simulink model "vtol_att_control"  (R2021a)
settings: Solver=FixedStepAuto  StartTime=0.0  StopTime=10.0  RelTol=1e-3
undefined symbols (not defined in the file): FW_PSP_OFF, MPC_XY_CRUISE, VT_ARSP_BLEND, VT_ARSP_TRANS, VT_B_DEC_FF, VT_B_DEC_I, VT_B_DEC_MSS, VT_B_REV_DEL, VT_B_REV_OUT, VT_B_TRANS_DUR, VT_B_TRANS_RAMP, VT_ELEV_MC_LOCK, VT_F_TRANS_THR, VT_FW_ALT_ERR, VT_FW_MIN_ALT, VT_FW_QC_P, VT_FW_QC_R, VT_PSHER_RMP_DT, VT_TRANS_MIN_TM, VT_TRANS_TIMEOUT
settings Model: DataDictionary=px4_dict.sldd  Creator=DELL  LastModifiedBy=DELL
settings OptimizationCC: GainParamInheritBuiltInType=on  UseFloatMulNetSlope=on  DefaultUnderspecifiedDataType=single  OptimizeBlockIOStorage=off  EnhancedBackFolding=on  PassReuseOutputArgsAs=Individual arguments  NoFixptDivByZeroProtection=on  EfficientFloat2IntCast=on  LifeSpan=1  OptimizeBlockOrder=speed  DifferentSizesBufferReuse=on  EfficientTunableParamExpr=on
settings DebuggingCC: ParameterTunabilityLossMsg=error
settings HardwareCC: ProdBitPerPointer=32  ProdBitPerSizeT=32  ProdBitPerPtrDiffT=32  ProdLargestAtomicInteger=Long  ProdLargestAtomicFloat=Double  ProdWordSize=32  ProdLongLongMode=on  ProdHWDeviceType=ARM Compatible->ARM Cortex-M
settings SFSimCC: MATLABDynamicMemAlloc=off
settings RTWCC: SystemTargetFile=ert.tlc  TemplateMakefile=ert_default_tmf  GenerateReport=on  LaunchReport=on  GenerateWebview=on  GenerateCodeMetricsReport=on
settings CodeAppCC: ForceParamTrailComments=on  IgnoreCustomStorageClasses=off  MaxIdLength=64  OperatorAnnotations=on  SimulinkDataObjDesc=on  SFDataObjDesc=on  MATLABFcnDesc=on  CustomSymbolStrGlobalVar=rt$N$M  CustomSymbolStrType=$N$M  CustomSymbolStrFcn=$N$M$F  CustomSymbolStrMacro=$N$M  InsertBlockDesc=on  SimulinkBlockComments=off  StateflowObjectComments=on
settings ERTTargetCC: TargetLangStandard=C99 (ISO)  GenerateSampleERTMain=on  CombineSignalStateStructs=on  SupportComplex=off  SupportNonInlinedSFcns=on  SupportVariableSizeSignals=on  RTWCAPISignals=on  RTWCAPIParams=on  RTWCAPIStates=on  ERTCustomFileTemplate=example_file_process.tlc  ERTFilePackagingFormat=CompactWithDataFile  IndentSize=4  MaxLineWidth=256

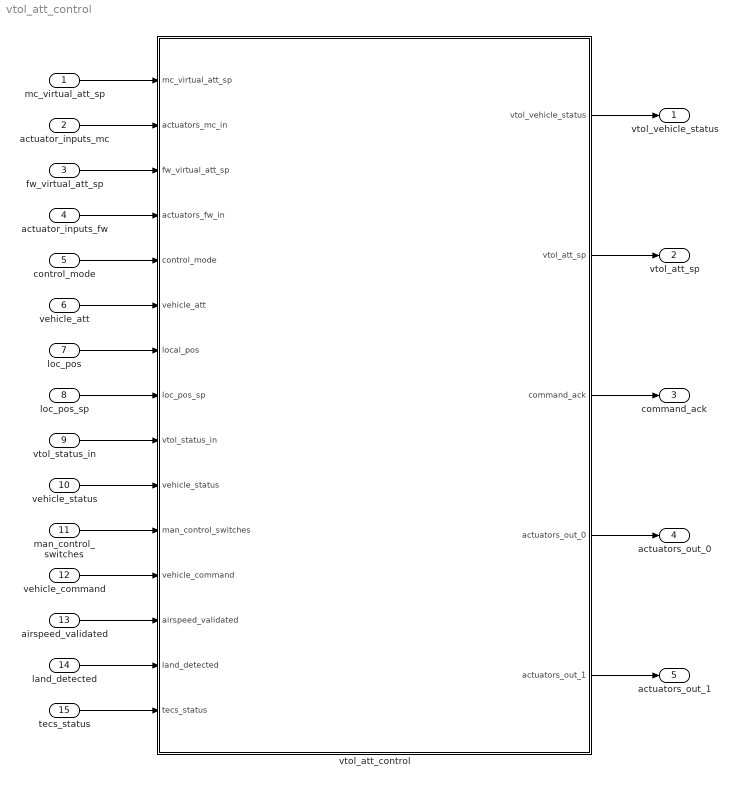
== system vtol_att_control ==
  mc_virtual_att_sp : Inport  OutDataTypeStr=Bus: px4_vehicle_attitude_setpoint  BusOutputAsStruct=on
  actuator_inputs_mc : Inport  Port=2  OutDataTypeStr=Bus: px4_actuator_controls_0  BusOutputAsStruct=on
  fw_virtual_att_sp : Inport  Port=3  OutDataTypeStr=Bus: px4_vehicle_attitude_setpoint  BusOutputAsStruct=on
  actuator_inputs_fw : Inport  Port=4  OutDataTypeStr=Bus: px4_actuator_controls_0  BusOutputAsStruct=on
  control_mode : Inport  Port=5  OutDataTypeStr=Bus: px4_vehicle_control_mode  BusOutputAsStruct=on
  vehicle_att : Inport  Port=6  OutDataTypeStr=Bus: px4_vehicle_attitude  BusOutputAsStruct=on
  loc_pos : Inport  Port=7  OutDataTypeStr=Bus: px4_vehicle_local_position  BusOutputAsStruct=on
  loc_pos_sp : Inport  Port=8  OutDataTypeStr=Bus: px4_vehicle_local_position_setpoint  BusOutputAsStruct=on
  vtol_status_in : Inport  Port=9  OutDataTypeStr=Bus: px4_vtol_vehicle_status  BusOutputAsStruct=on
  vehicle_status : Inport  Port=10  OutDataTypeStr=Bus: px4_vehicle_status  BusOutputAsStruct=on
  man_control_switches : Inport  Port=11  OutDataTypeStr=Bus: px4_manual_control_switches  BusOutputAsStruct=on
  vehicle_command : Inport  Port=12  OutDataTypeStr=Bus: px4_vehicle_command  BusOutputAsStruct=on
  airspeed_validated : Inport  Port=13  OutDataTypeStr=Bus: px4_airspeed_validated  BusOutputAsStruct=on
  land_detected : Inport  Port=14  OutDataTypeStr=Bus: px4_vehicle_land_detected  BusOutputAsStruct=on
  tecs_status : Inport  Port=15  OutDataTypeStr=Bus: px4_tecs_status  BusOutputAsStruct=on
  vtol_att_control : Stateflow chart  TreatAsAtomicUnit=on
  vtol_vehicle_status : Outport  OutDataTypeStr=Bus: px4_vtol_vehicle_status
  vtol_att_sp : Outport  Port=2  OutDataTypeStr=Bus: px4_vehicle_attitude_setpoint
  command_ack : Outport  Port=3  OutDataTypeStr=Bus: px4_vehicle_command_ack
  actuators_out_0 : Outport  Port=4  OutDataTypeStr=Bus: px4_actuator_controls_0
  actuators_out_1 : Outport  Port=5  OutDataTypeStr=Bus: px4_actuator_controls
  wires:
  fw_virtual_att_sp/1 -> vtol_att_control/3(fw_virtual_att_sp)
  actuator_inputs_mc/1 -> vtol_att_control/2(actuators_mc_in)
  vehicle_att/1 -> vtol_att_control/6(vehicle_att)
  loc_pos/1 -> vtol_att_control/7(local_pos)
  vehicle_command/1 -> vtol_att_control/12(vehicle_command)
  airspeed_validated/1 -> vtol_att_control/13(airspeed_validated)
  control_mode/1 -> vtol_att_control/5(control_mode)
  mc_virtual_att_sp/1 -> vtol_att_control/1(mc_virtual_att_sp)
  vtol_att_control/4(actuators_out_0) -> actuators_out_0/1
  loc_pos_sp/1 -> vtol_att_control/8(loc_pos_sp)
  land_detected/1 -> vtol_att_control/14(land_detected)
  actuator_inputs_fw/1 -> vtol_att_control/4(actuators_fw_in)
  tecs_status/1 -> vtol_att_control/15(tecs_status)
  vtol_att_control/2(vtol_att_sp) -> vtol_att_sp/1
  vtol_att_control/3(command_ack) -> command_ack/1
  vtol_att_control/1(vtol_vehicle_status) -> vtol_vehicle_status/1
  vtol_status_in/1 -> vtol_att_control/9(vtol_status_in)
  vehicle_status/1 -> vtol_att_control/10(vehicle_status)
  vtol_att_control/5(actuators_out_1) -> actuators_out_1/1
  man_control_switches/1 -> vtol_att_control/11(man_control_switches)

== stateflow chart vtol_att_control/vtol_att_control ==
  state vehicle_cmd_poll [parallel]
    settings: executionOrder=1
    state DO_VTOL_TRANSITION
      en:
      result = PX4_VEHICLE_COMMAND_ACK.VEHICLE_RESULT_ACCEPTED;
      % 在自动起飞阶段、或者在land或者RTL模式下拒绝从RW转换到FW
      if (vehicle_command.command == PX4_VEHICLE_COMMAND.VEHICLE_CMD_DO_VTOL_TRANSITION)
      if (vehicle_status.nav_state == PX4_VEHICLE_STATUS.NAVIGATION_STATE_AUTO_TAKEOFF || ...
      (vehicle_status.vehicle_type == PX4_VEHICLE_STATUS.VEHICLE_TYPE_ROTARY_WING && ...
      vehicle_status.nav_state == PX4_VEHICLE_STATUS.NAVIGATION_STATE_AUTO_LAND || ...
      vehicle_status.nav_state == PX4_VEHICLE_STATUS.NAVIGATION_STATE_AUTO_RTL))
      result = PX4_VEHICLE_COMMAND_ACK.VEHICLE_RESULT_TEMPORARILY_REJECTED;
      else
      transition_command_ = int8(vehicle_command.param1 + 0.5);
      if (isfinite(vehicle_command.param2))
      immediate_transition_ = int8(vehicle_command.param2 + 0.5)
      else
      immediate_transition_ = int8(false);
      end
      end
      end
      % 如果command是来自外部的，不是飞机自己发布的
      if (vehicle_command.from_external)
      command_ack.timestamp = uint64(getSimulationTime * 1e+6); % 单位：us
      command_ack.command = vehicle_command.command;
      command_ack.result = uint8(result);
      command_ack.target_system = vehicle_command.source_system;
      command_ack.target_component = vehicle_command.source_component;
      end
    state NONE
    state KEEP_IN_MC
      en:
      transition_command_ = int8(PX4_VTOL_VEHICLE_STATUS.VEHICLE_VTOL_STATE_MC);
    state KEEP_IN_FW
      en:
      transition_command_ = int8(PX4_VTOL_VEHICLE_STATUS.VEHICLE_VTOL_STATE_FW);
    state TRANSITION_TO_MC
      en:
      % We want to make sure that a mode change (manual>auto) during the back transition
      % doesn't result in an unsafe state. This prevents the instant fall back to
      % fixed-wing on the switch from manual to auto.
      % 飞机本来是在从固定翼过渡到旋翼模式的时候，如果接管，那么直接变成旋翼模式
      transition_command_ = int8(PX4_VTOL_VEHICLE_STATUS.VEHICLE_VTOL_STATE_MC);
    state NONE1
    (default) -> (junction 580)
    vehicle_cmd_poll -> (junction 580) [order 1] : % 轮询是否有开启转换的指令
        | [hasChanged(vehicle_command.timestamp)]
    (junction 580) -> DO_VTOL_TRANSITION [order 1] : [vehicle_command.command == PX4_VEHICLE_COMMAND.VEHICLE_CMD_DO_VTOL_TRANSITION]
    (junction 580) -> (junction 581) [order 2]
    (junction 581) -> NONE
    vehicle_cmd_poll -> (junction 582) [order 2] : % reset transition command if not auto control
        | [control_mode.flag_control_manual_enabled == true]
    (junction 582) -> KEEP_IN_MC [order 1] : % vtol_mode_ == mode::ROTARY_WING
        | [vtol_mode_ == uint8(3)]
    (junction 582) -> (junction 583) [order 2]
    (junction 583) -> KEEP_IN_FW [order 1] : % vtol_mode_ == mode::FIXED_WING
        | [vtol_mode_ == uint8(4)]
    (junction 583) -> (junction 584) [order 2]
    (junction 584) -> TRANSITION_TO_MC [order 1] : % mode::TRANSITION_TO_MC
        | [vtol_mode_ == uint8(2)]
    (junction 584) -> (junction 585) [order 2]
    (junction 585) -> NONE1
  state vtol_state_flow [parallel]
    settings: executionOrder=2
    state MC_MODE_
      en:
      vtol_schedule_.flight_mode = uint8(PX4_VTOL_MODE.MC_MODE);
      vtol_mode_ = uint8(PX4_VTOL_MODETYPE.ROTARY_WING);
      % 转换失败保护或者没有开启过渡到固定翼的开关，那么启用旋翼模式
      if (vtol_status_in.vtol_transition_failsafe || ~vtol_state_flow.is_fixed_wing_requested)
      pusher_throttle_ = single(0.0);
      reverse_output_ = single(0.0);
      % reset failsafe when FW is no longer requested
      % 转换失败后，如果转换通道还在保持请求转换到固定翼，那么vtol_transition_failsafe标志位保持置位为true
      % 转换失败后，用户不再请求转换到固定翼，vtol_transition_failsafe标志位重置为false
      if (vtol_status_in.vtol_transition_failsafe && ~vtol_state_flow.is_fixed_wing_requested)
      vtol_vehicle_status.vtol_transition_failsafe = false;
      end
      end
      % 正常进入，关闭固定翼转换
      en,du:
      mc_weight_ = single(1.0);
      pusher_throttle_ = single(0.0);
      reverse_output_ = single(0.0);
      %
      % update mc mode
      vtol_vehicle_status.vtol_in_rw_mode = true;
      vtol_vehicle_status.vtol_in_trans_mode = false;
      vtol_vehicle_status.in_transition_to_fw = false;
      if (~flag_idle_mc_)
      % flag_idle_mc_ = set_idle_mc();
      end
      % resetAccelToPitchPitchIntegrator
      accel_to_pitch_integ_ = single(0.0);
      % mode_action.set_all_motor_state(PX4_MOTOR_STATE.ENABLED, 0);
      mc_roll_weight_ = 1.0;
      mc_pitch_weight_ = 1.0;
      mc_yaw_weight_ = 1.0;
      mc_throttle_weight_ = 1.0;
      % pusher_assist()没看懂这个函数
      % publish actuators_out_0
      vtol_att_sp = mc_virtual_att_sp;
      elevon_lock = (VT_ELEV_MC_LOCK == 1);
      now_us = uint64(getSimulationTime * 1e+6);
      actuators_out_0.timestamp = now_us;
      actuators_out_0.timestamp_sample = actuators_mc_in.timestamp_sample;
      actuators_out_0.control(PX4_ACTUATOR_CONTROLS.INDEX_ROLL) = actuators_mc_in.control(PX4_ACTUATOR_CONTROLS.INDEX_ROLL);
      actuators_out_0.control(PX4_ACTUATOR_CONTROLS.INDEX_PITCH) = actuators_mc_in.control(PX4_ACTUATOR_CONTROLS.INDEX_PITCH);
      actuators_out_0.control(PX4_ACTUATOR_CONTROLS.INDEX_YAW) = actuators_mc_in.control(PX4_ACTUATOR_CONTROLS.INDEX_YAW);
      actuators_out_0.control(PX4_ACTUATOR_CONTROLS.INDEX_THROTTLE) = actuators_mc_in.control(PX4_ACTUATOR_CONTROLS.INDEX_THROTTLE);
      actuators_out_0.control(PX4_ACTUATOR_CONTROLS.INDEX_LANDING_GEAR) = actuators_mc_in.control(PX4_ACTUATOR_CONTROLS.INDEX_LANDING_GEAR);
      % publish actuators_out_1
      actuators_out_1.timestamp = now_us;
      actuators_out_1.timestamp_sample = actuators_mc_in.timestamp_sample;
      actuators_out_1.control(PX4_ACTUATOR_CONTROLS.INDEX_ROLL) = single(~elevon_lock) * actuators_fw_in.control(PX4_ACTUATOR_CONTROLS.INDEX_ROLL);
      actuators_out_1.control(PX4_ACTUATOR_CONTROLS.INDEX_PITCH) = single(~elevon_lock) * actuators_fw_in.control(PX4_ACTUATOR_CONTROLS.INDEX_PITCH);
      actuators_out_1.control(PX4_ACTUATOR_CONTROLS.INDEX_YAW) = single(0.0);
      actuators_out_1.control(PX4_ACTUATOR_CONTROLS.INDEX_THROTTLE) = pusher_throttle_;
      actuators_out_1.control(PX4_ACTUATOR_CONTROLS.INDEX_FLAPS) = single(0.0);
      actuators_out_1.control(PX4_ACTUATOR_CONTROLS.INDEX_AIRBRAKES) = single(0.0);
    state TRANSITION_TO_FW_
      en:
      vtol_schedule_.transition_start = uint64(getSimulationTime) * 1e+6; % 单位：us
      vtol_schedule_.flight_mode = uint8(PX4_VTOL_MODE.TRANSITION_TO_FW);
      vtol_mode_ = uint8(PX4_VTOL_MODETYPE.TRANSITION_TO_FW);
      % 飞机当前正处于过渡到固定翼的阶段
      en,du:
      % 计算转换条件（看是否能转换到固定翼阶段）
      time_since_trans_start_ = single(elapsed(sec));
      % update transition to fw
      vtol_vehicle_status.vtol_in_trans_mode = true;
      vtol_vehicle_status.vtol_in_rw_mode = true; % making mc attitude controller work during transition
      vtol_vehicle_status.in_transition_to_fw = (vtol_mode_ == PX4_VTOL_MODETYPE.TRANSITION_TO_FW);
      %
      if ((flag_was_in_trans_mode_ == false) || hasChanged(mc_virtual_att_sp.timestamp) || hasChanged(fw_virtual_att_sp.timestamp))
      vtol_state_flow.check_quadchute_condition;
      % copy virtual attitude setpoint to real attitude setpoint
      vtol_att_sp = mc_virtual_att_sp;
      transition_to_fw;
      % publish actuators_out_0
      now_us = uint64(getSimulationTime * 1e+6);
      actuators_out_0.timestamp = now_us;
      actuators_out_0.timestamp_sample = actuators_mc_in.timestamp_sample;
      actuators_out_0.control(PX4_ACTUATOR_CONTROLS.INDEX_ROLL) = actuators_mc_in.control(PX4_ACTUATOR_CONTROLS.INDEX_ROLL) * mc_roll_weight_;
      actuators_out_0.control(PX4_ACTUATOR_CONTROLS.INDEX_PITCH) = actuators_mc_in.control(PX4_ACTUATOR_CONTROLS.INDEX_PITCH) * mc_pitch_weight_;
      actuators_out_0.control(PX4_ACTUATOR_CONTROLS.INDEX_YAW) = actuators_mc_in.control(PX4_ACTUATOR_CONTROLS.INDEX_YAW) * mc_yaw_weight_;
      actuators_out_0.control(PX4_ACTUATOR_CONTROLS.INDEX_THROTTLE) = actuators_mc_in.control(PX4_ACTUATOR_CONTROLS.INDEX_THROTTLE) * mc_throttle_weight_;
      actuators_out_0.control(PX4_ACTUATOR_CONTROLS.INDEX_LANDING_GEAR) = single(0.0);
      % publish actuators_out_1
      actuators_out_1.timestamp = now_us;
      actuators_out_1.timestamp_sample = actuators_mc_in.timestamp_sample;
      actuators_out_1.control(PX4_ACTUATOR_CONTROLS.INDEX_ROLL) = actuators_fw_in.control(PX4_ACTUATOR_CONTROLS.INDEX_ROLL);
      actuators_out_1.control(PX4_ACTUATOR_CONTROLS.INDEX_PITCH) = actuators_fw_in.control(PX4_ACTUATOR_CONTROLS.INDEX_PITCH);
      actuators_out_1.control(PX4_ACTUATOR_CONTROLS.INDEX_YAW) = actuators_fw_in.control(PX4_ACTUATOR_CONTROLS.INDEX_YAW);
      actuators_out_1.control(PX4_ACTUATOR_CONTROLS.INDEX_THROTTLE) = pusher_throttle_;
      actuators_out_1.control(PX4_ACTUATOR_CONTROLS.INDEX_FLAPS) = actuators_fw_in.control(PX4_ACTUATOR_CONTROLS.INDEX_FLAPS);
      actuators_out_1.control(PX4_ACTUATOR_CONTROLS.INDEX_AIRBRAKES) = reverse_output_;
      end
    state FW_MODE_
      en:
      trans_finished_ts_ = uint64(getSimulationTime * 1e+6); % 单位：us
      vtol_schedule_.flight_mode = uint8(PX4_VTOL_MODE.FW_MODE);
      vtol_mode_ = uint8(PX4_VTOL_MODETYPE.FIXED_WING);
      % 正常情况下，进入固定翼模式后，保持该模式飞行
      en,du:
      mc_weight_ = single(0.0);
      vtol_vehicle_status.vtol_in_rw_mode = false;
      vtol_vehicle_status.vtol_in_trans_mode = false;
      vtol_vehicle_status.in_transition_to_fw = false;
      % 更新固定翼状态
      if (hasChanged(fw_virtual_att_sp.timestamp))
      if (flag_idle_mc_)
      % flag_idle_mc_ = ~set_idle_fw();
      end
      % resetAccelToPitchPitchIntegrator
      accel_to_pitch_integ_ = single(0.0);
      % set_alternate_motor_state(PX4_MOTOR_STATE.DISABLED, 0);
      mc_roll_weight_ = single(0.0);
      mc_pitch_weight_ = single(0.0);
      mc_yaw_weight_ = single(0.0);
      %
      % publish
      % copy virtual attitude setpoint to real attitude setpoint
      vtol_att_sp = fw_virtual_att_sp;
      % 在转换成固定翼完成后，tecs还未发布tecs_status的topic，暂时“认为”tecs没有running
      if (tecs_status.timestamp < trans_finished_ts_)
      tecs_running_ = false;
      elseif (~tecs_running_)
      tecs_running_ = true;
      tecs_running_ts = uint64(getSimulationTime) * 1e+6; % 单位：us
      end
      % 如果tecs没有运行，或在手动控制高度的情况下，tecs发布了但控制器还没运行完，保持pusher_throttle_不变
      if((~tecs_running_ || (tecs_running_ && fw_virtual_att_sp.timestamp <= tecs_running_ts)) && control_mode.flag_control_altitude_enabled)
      % keep thrust from transition
      vtol_att_sp.thrust_body(1) = pusher_throttle_;
      end
      vtol_state_flow.check_quadchute_condition;
      % publish actuators_out_0
      actuators_out_0.timestamp = now_us;
      actuators_out_0.timestamp_sample = actuators_mc_in.timestamp_sample;
      actuators_out_0.control(PX4_ACTUATOR_CONTROLS.INDEX_ROLL) = single(0.0);
      actuators_out_0.control(PX4_ACTUATOR_CONTROLS.INDEX_PITCH) = single(0.0);
      actuators_out_0.control(PX4_ACTUATOR_CONTROLS.INDEX_YAW) = single(0.0);
      actuators_out_0.control(PX4_ACTUATOR_CONTROLS.INDEX_THROTTLE) = single(0.0);
      actuators_out_0.control(PX4_ACTUATOR_CONTROLS.INDEX_LANDING_GEAR) = single(0.0);
      % publish actuators_out_1
      actuators_out_1.timestamp = now_us;
      actuators_out_1.timestamp_sample = actuators_mc_in.timestamp_sample;
      actuators_out_1.control(PX4_ACTUATOR_CONTROLS.INDEX_ROLL) = actuators_fw_in.control(PX4_ACTUATOR_CONTROLS.INDEX_ROLL);
      actuators_out_1.control(PX4_ACTUATOR_CONTROLS.INDEX_PITCH) = actuators_fw_in.control(PX4_ACTUATOR_CONTROLS.INDEX_PITCH);
      actuators_out_1.control(PX4_ACTUATOR_CONTROLS.INDEX_YAW) = actuators_fw_in.control(PX4_ACTUATOR_CONTROLS.INDEX_YAW);
      actuators_out_1.control(PX4_ACTUATOR_CONTROLS.INDEX_THROTTLE) = actuators_fw_in.control(PX4_ACTUATOR_CONTROLS.INDEX_THROTTLE);
      actuators_out_1.control(PX4_ACTUATOR_CONTROLS.INDEX_FLAPS) = actuators_fw_in.control(PX4_ACTUATOR_CONTROLS.INDEX_FLAPS);
      actuators_out_1.control(PX4_ACTUATOR_CONTROLS.INDEX_AIRBRAKES) = actuators_fw_in.control(PX4_ACTUATOR_CONTROLS.INDEX_LANDING_GEAR);
      end
    state TRANSITION_TO_MC_
      en:
      % 没有请求转换到固定翼模式，就会切回旋翼模式
      if (~vtol_state_flow.is_fixed_wing_requested)
      % 单位：us
      vtol_schedule_.transition_start = uint64(getSimulationTime * 1e+6);
      reverse_output_ = constrain(VT_B_REV_OUT, 0.0, 1.0);
      end
      % 固定翼转多旋翼
      en,du:
      % 计算转换成旋翼模式失败的条件
      time_since_trans_start_ = single(elapsed(sec));
      R_to_body = quat_to_dcm(vehicle_att.q);
      vel = R_to_body * [local_pos.vx; local_pos.vy; local_pos.vz];
      x_vel = vel(1);
      % 更新过渡转换，转换到多旋翼模式
      vtol_vehicle_status.vtol_in_trans_mode = true;
      vtol_vehicle_status.vtol_in_rw_mode = true;
      vtol_vehicle_status.in_transition_to_fw = (vtol_mode_ == PX4_VTOL_MODETYPE.TRANSITION_TO_FW);
      transition_to_mc();
      % publish actuators_out_0
      now_us = uint64(getSimulationTime * 1e+6);
      actuators_out_0.timestamp = now_us;
      actuators_out_0.timestamp_sample = actuators_mc_in.timestamp_sample;
      actuators_out_0.control(PX4_ACTUATOR_CONTROLS.INDEX_ROLL) = actuators_mc_in.control(PX4_ACTUATOR_CONTROLS.INDEX_ROLL) * mc_roll_weight_;
      actuators_out_0.control(PX4_ACTUATOR_CONTROLS.INDEX_PITCH) = actuators_mc_in.control(PX4_ACTUATOR_CONTROLS.INDEX_PITCH) * mc_pitch_weight_;
      actuators_out_0.control(PX4_ACTUATOR_CONTROLS.INDEX_YAW) = actuators_mc_in.control(PX4_ACTUATOR_CONTROLS.INDEX_YAW) * mc_yaw_weight_;
      actuators_out_0.control(PX4_ACTUATOR_CONTROLS.INDEX_THROTTLE) = actuators_mc_in.control(PX4_ACTUATOR_CONTROLS.INDEX_THROTTLE) * mc_throttle_weight_;
      actuators_out_0.control(PX4_ACTUATOR_CONTROLS.INDEX_LANDING_GEAR) = single(0.0);
      % publish actuators_out_1
      actuators_out_1.timestamp = now_us;
      actuators_out_1.timestamp_sample = actuators_mc_in.timestamp_sample;
      actuators_out_1.control(PX4_ACTUATOR_CONTROLS.INDEX_ROLL) = actuators_fw_in.control(PX4_ACTUATOR_CONTROLS.INDEX_ROLL);
      actuators_out_1.control(PX4_ACTUATOR_CONTROLS.INDEX_PITCH) = actuators_fw_in.control(PX4_ACTUATOR_CONTROLS.INDEX_PITCH);
      actuators_out_1.control(PX4_ACTUATOR_CONTROLS.INDEX_YAW) = actuators_fw_in.control(PX4_ACTUATOR_CONTROLS.INDEX_YAW);
      actuators_out_1.control(PX4_ACTUATOR_CONTROLS.INDEX_THROTTLE) = pusher_throttle_;
      actuators_out_1.control(PX4_ACTUATOR_CONTROLS.INDEX_FLAPS) = actuators_fw_in.control(PX4_ACTUATOR_CONTROLS.INDEX_FLAPS);
      actuators_out_1.control(PX4_ACTUATOR_CONTROLS.INDEX_AIRBRAKES) = reverse_output_;
    (default) -> MC_MODE_
    MC_MODE_ -> TRANSITION_TO_FW_ : % 请求转换到固定翼模式
        | [is_fixed_wing_requested()]
    TRANSITION_TO_FW_ -> FW_MODE_ [order 1] : % 满足转换时间且空速大于转换的阈值
        | % 或未解锁或飞机在地面
        | [((time_since_trans_start_ > VT_TRANS_MIN_TM) && ...
        | isfinite(airspeed_validated.calibrated_airspeed_m_s) && ...
        | (airspeed_validated.calibrated_airspeed_m_s >= VT_TRANS_MIN_TM)) || ...
        | (~control_mode.flag_armed || land_detected.landed)]
    TRANSITION_TO_FW_ -> MC_MODE_ [order 2] : % 没有请求转换到固定翼模式
        | % 或者转换失败
        | [~is_fixed_wing_requested() || ...
        | vtol_status_in.vtol_transition_failsafe]
    (junction 533) -> MC_MODE_
    TRANSITION_TO_MC_ -> TRANSITION_TO_FW_ [order 1] : % 请求转换到固定翼模式
        | [is_fixed_wing_requested()]
    FW_MODE_ -> (junction 537)
    TRANSITION_TO_MC_ -> (junction 533) [order 2] : % 转换超时，或者前向速度低于旋翼的巡航速
        | % 或未解锁或飞机在地面
        | [(time_since_trans_start_ > VT_B_TRANS_DUR) || ...
        |  (local_pos.v_xy_valid && x_vel <= MPC_XY_CRUISE) || ...
        |  (~control_mode.flag_armed || land_detected.landed)]
    (junction 537) -> TRANSITION_TO_MC_ : % 没有请求转换到固定翼模式
        | [~is_fixed_wing_requested() || ...
        | (vtol_schedule_.flight_mode == uint8(PX4_VTOL_MODE.TRANSITION_TO_MC))]
  data: result local Enum: PX4_VEHICLE_COMMAND_ACK size=1; to_fw function_output; elevon_lock local boolean size=1 =false; tecs_running_ts local uint64 size=1 =uint64(0); R_to_body local single size=[3 3]; vel local single size=[3 1]; x_vel local single size=1 =single(0.0); quadchute_command_treated_ local boolean size=1 =false; tecs_running_ local boolean size=1 =false; ra_hrate_ local single size=1 =single(0.0); ra_hrate_sp_ local single size=1 =single(0.0); now_us local uint64 size=1 =uint64(0); mc_virtual_att_sp input Bus: px4_vehicle_attitude_setpoint size=1; actuators_mc_in input Bus: px4_actuator_controls_0 size=1; fw_virtual_att_sp input Bus: px4_vehicle_attitude_setpoint size=1; actuators_fw_in input Bus: px4_actuator_controls_0 size=1; control_mode input Bus: px4_vehicle_control_mode size=1; vehicle_att input Bus: px4_vehicle_attitude size=1; local_pos input Bus: px4_vehicle_local_position size=1; loc_pos_sp input Bus: px4_vehicle_local_position_setpoint size=1; vtol_status_in input Bus: px4_vtol_vehicle_status size=1; vehicle_status input Bus: px4_vehicle_status size=1; man_control_switches input Bus: px4_manual_control_switches size=1; vehicle_command input Bus: px4_vehicle_command size=1; pusher_throttle_ local single size=1 =single(0.0); reverse_output_ local single size=1 =single(0.0); vtol_vehicle_status output Bus: px4_vtol_vehicle_status size=1; vtol_schedule_ local Bus: px4_vtol_schedule size=1; mc_weight_ local single size=1 =single(1.0); VT_B_REV_OUT parameter size=1; airspeed_validated input Bus: px4_airspeed_validated size=1; VT_TRANS_MIN_TM parameter size=1; VT_ARSP_TRANS parameter size=1; trans_finished_ts_ local uint64 size=1 =uint64(0); vtol_mode_ local uint8 size=1 =uint8(3); transition_command_ local int8 size=1 =int8(3); VT_PSHER_RMP_DT parameter size=1; VT_F_TRANS_THR parameter size=1; VT_ARSP_BLEND parameter size=1; vtol_att_sp output Bus: px4_vehicle_attitude_setpoint size=1; command_ack output Bus: px4_vehicle_command_ack size=1; FW_PSP_OFF parameter size=1; VT_TRANS_TIMEOUT parameter size=1; VT_B_REV_DEL parameter size=1; VT_B_TRANS_RAMP parameter size=1; flag_idle_mc_ local boolean size=1 =false; mc_roll_weight_ local single size=1 =single(0.0); mc_pitch_weight_ local single size=1 =single(0.0); mc_yaw_weight_ local single size=1 =single(0.0); mc_throttle_weight_ local single size=1 =single(0.0); VT_B_DEC_MSS parameter size=1; VT_B_DEC_FF parameter size=1; accel_to_pitch_integ_ local single size=1 =single(0.0); VT_B_DEC_I parameter size=1; actuators_out_0 output Bus: px4_actuator_controls_0 size=1; actuators_out_1 output Bus: px4_actuator_controls size=1; VT_ELEV_MC_LOCK parameter size=1; MPC_XY_CRUISE parameter size=1; land_detected input Bus: px4_vehicle_land_detected size=1; VT_B_TRANS_DUR parameter size=1; time_since_trans_start_ local single size=1 =single(0.0); flag_was_in_trans_mode_ local boolean size=1 =false; immediate_transition_ local int8 size=1 =int8(0); VT_FW_MIN_ALT parameter size=1; VT_FW_ALT_ERR parameter size=1; tecs_status input Bus: px4_tecs_status size=1; VT_FW_QC_P parameter size=1; VT_FW_QC_R parameter size=1
  data x_vel settings: description=this is my var
  data transition_command_ settings: description=|
      | static constexpr uint8_t VEHICLE_VTOL_STATE_UNDEFINED = 0;
      | static constexpr uint8_t VEHICLE_VTOL_STATE_TRANSITION_TO_FW = 1;
      | static constexpr uint8_t VEHICLE_VTOL_STATE_TRANSITION_TO_MC = 2;
      | static constexpr uint8_t VEHICLE_VTOL_STATE_MC = 3;
      | static constexpr uint8_t VEHICLE_VTOL_STATE_FW = 4;
  function to_fw = is_fixed_wing_requested:
    | % Returns true if fixed-wing mode is requested. Changed either via switch or via command.
    | function to_fw = is_fixed_wing_requested
    | 
    | to_fw = false;
    | 
    | if (man_control_switches.transition_switch ~= PX4_MANUAL_CONTROL_SWITCHES.SWITCH_POS_NONE && ...
    |         control_mode.flag_control_manual_enabled)
    |     
    |     % 判断飞手是否想要切换到FW模式
    |     to_fw = (man_control_switches.transition_switch == PX4_MANUAL_CONTROL_SWITCHES.SWITCH_POS_ON);
    |     
    | else
    |     
    |     % listen to transition commands if not in manual or mode switch is not mapped
    |     % 判断地面站是否想要切换到FW模式
    |     to_fw = (transition_command_ == PX4_VTOL_VEHICLE_STATUS.VEHICLE_VTOL_STATE_FW);
    |     
    | end
    | 
    | end
  function check_quadchute_condition:
    | %% QuadChute Altitude
    | %
    | % Minimum altitude for fixed wing flight, when in fixed wing the altitude drops below this altitude
    | % the vehicle will transition back to MC mode and enter failsafe RTL
    | % @min 0.0
    | % @max 200.0
    | % @group VTOL Attitude Control
    | % PARAM_DEFINE_FLOAT(VT_FW_MIN_ALT, 0.0f);
    | 
    | %% Adaptive QuadChute
    | %
    | % Maximum negative altitude error for fixed wing flight. If the altitude drops below this value below the altitude setpoint
    | % the vehicle will transition back to MC mode and enter failsafe RTL.
    | % @min 0.0
    | % @max 200.0
    | % @group VTOL Attitude Control
    | % PARAM_DEFINE_FLOAT(VT_FW_ALT_ERR, 0.0f);
    | 
    | %% QuadChute Max Pitch
    | %
    | % Maximum pitch angle before QuadChute engages
    | % Above this the vehicle will transition back to MC mode and enter failsafe RTL
    | % @min 0
    | % @max 180
    | % @group VTOL Attitude Control
    | % PARAM_DEFINE_INT32(VT_FW_QC_P, 0);
    | 
    | %% QuadChute Max Roll
    | %
    | % Maximum roll angle before QuadChute engages
    | % Above this the vehicle will transition back to MC mode and enter failsafe RTL
    | % @min 0
    | % @max 180
    | % @group VTOL Attitude Control
    | % PARAM_DEFINE_INT32(VT_FW_QC_R, 0);
    | 
    | %% Checks for fixed-wing failsafe condition and issues abort request if needed.
    | function check_quadchute_condition
    | 
    | %% 如果收到立即转换到旋翼模式的命令，立即转换
    | if ((transition_command_ == int8(PX4_VTOL_VEHICLE_STATUS.VEHICLE_VTOL_STATE_MC)) && ...
    |         (immediate_transition_ == true) && (quadchute_command_treated_ == false))
    |     if (vtol_vehicle_status.vtol_transition_failsafe == false)
    |         sprintf("QuadChute by external command")
    |         vtol_vehicle_status.vtol_transition_failsafe = true;
    |     end
    |     quadchute_command_treated_ = true;
    |     immediate_transition_ = int8(false);
    | else
    |     quadchute_command_treated_ = false;
    | end
    | 
    | %% reset the filtered height rate and heigh rate setpoint if TECS is not running
    | if (~tecs_running_)
    |     ra_hrate_ = single(0.0);
    |     ra_hrate_sp_ = single(0.0);
    | end
    | 
    | %% 飞机已经解锁且没有着陆
    | if (control_mode.flag_armed && ~land_detected.landed)
    |     
    |     %% 计算欧拉角
    |     eulZYX = quat2eul(vehicle_att.q', 'ZYX');
    |     phi = eulZYX(3);
    |     theta = eulZYX(2);
    |     psi = eulZYX(1);
    |     
    |     %% fixed-wing minimum altitude
    |     if ((VT_FW_MIN_ALT > eps) && (-local_pos.z < VT_FW_MIN_ALT))
    |         if (vtol_vehicle_status.vtol_transition_failsafe == false)
    |             sprintf("QuadChute: Minimum altitude breached")
    |             vtol_vehicle_status.vtol_transition_failsafe = true;
    |         end
    |     end
    |     
    |     %% adaptive quadchute
    |     if ((VT_FW_ALT_ERR > eps) && (control_mode.flag_control_altitude_enabled))
    |         % 在过渡阶段使用tecs控制固定翼，主要检查高度误差以及高程速率误差是否过大
    |         % We use tecs for tracking in FW and loc_pos_sp during transitions
    |         if (tecs_running_)
    |             % 1 second rolling average
    |             ra_hrate_ = (49 * ra_hrate_ + tecs_status.height_rate) / 50;
    |             ra_hrate_sp_ = (49 * ra_hrate_sp_ + tecs_status.height_rate_setpoint) / 50;
    |             
    |             % are we dropping while requesting significant ascend?
    |             if (((tecs_status.altitude_sp - tecs_status.altitude_filtered) > VT_FW_ALT_ERR) && (ra_hrate_ < -1.0) && (ra_hrate_sp_ > 1.0))
    |                 if (vtol_vehicle_status.vtol_transition_failsafe == false)
    |                     sprintf("QuadChute: loss of altitude")
    |                     vtol_vehicle_status.vtol_transition_failsafe = true;
    |                 end
    |             else
    |                 height_error = local_pos.z_valid && ((-loc_pos_sp.z - -local_pos.z) > VT_FW_ALT_ERR);
    |                 height_rate_error = local_pos.v_z_valid && (local_pos.vz > 1.0) && (local_pos.z_deriv > 1.0);
    |                 if (height_error && height_rate_error)
    |                     if (vtol_vehicle_status.vtol_transition_failsafe == false)
    |                         sprintf("QuadChute: large altitude error")
    |                         vtol_vehicle_status.vtol_transition_failsafe = true;
    |                     end
    |                 end
    |             end
    |         end
    |         
    |         %% fixed-wing maximum pitch angle
    |         if (VT_FW_QC_P > 0.0)
    |             if (theta > abs(deg2rad(single(VT_FW_QC_P))))
    |                 if (vtol_vehicle_status.vtol_transition_failsafe == false)
    |                     sprintf("Maximum pitch angle exceeded")
    |                     vtol_vehicle_status.vtol_transition_failsafe = true;
    |                 end
    |             end
    |         end
    |         
    |         %% fixed-wing maximum roll angle
    |         if (VT_FW_QC_R > 0)
    |             if (phi > abs(deg2rad(single(VT_FW_QC_R))))
    |                 if (vtol_vehicle_status.vtol_transition_failsafe == false)
    |                     sprintf("Maximum pitch angle exceeded")
    |                     vtol_vehicle_status.vtol_transition_failsafe = true;
    |                 end
    |             end
    |         end
    |         
    |     end
    |     
    | end
    | 
    | end
  function transition_to_fw:
    | %% VT_PSHER_RMP_DT
    | % Defines the time window during which the pusher throttle will be ramped up linearly to VT_F_TRANS_THR during a transition
    | % to fixed wing mode. Zero or negative values will produce an instant throttle rise to VT_F_TRANS_THR.
    | % @max 20
    | % @increment 0.01
    | % @decimal 2
    | % @group VTOL Attitude Control
    | % PARAM_DEFINE_FLOAT(VT_PSHER_RMP_DT, 3.0f);
    | 
    | %% VT_F_TRANS_THR
    | % Target throttle value for the transition to fixed wing flight.
    | % standard vtol: pusher
    | % tailsitter, tiltrotor: main throttle
    | % @min 0.0
    | % @max 1.0
    | % @increment 0.01
    | % @decimal 3
    | % @group VTOL Attitude Control
    | % PARAM_DEFINE_FLOAT(VT_F_TRANS_THR, 1.0f);
    | 
    | %% FW_PSP_OFF
    | % Pitch setpoint offset (pitch at level flight)
    | % An airframe specific offset of the pitch setpoint in degrees, the value is
    | % added to the pitch setpoint and should correspond to the pitch at
    | % typical cruise speed of the airframe.
    | % @unit deg
    | % @min -90.0
    | % @max 90.0
    | % @decimal 1
    | % @increment 0.5
    | % @group FW Attitude Control
    | 
    | %% -----------------------------------------------------------------------------------------------------
    | function transition_to_fw
    | 
    | %% 计算pusher_throttle_
    | % 参数VT_PSHER_RMP_DT小于0，油门立即搞到最大；否则，油门在VT_PSHER_RMP_DT内线性增加到最大值
    | if (VT_PSHER_RMP_DT < 0.0)
    |     pusher_throttle_ = VT_F_TRANS_THR;
    | else
    |     pusher_throttle_ = VT_F_TRANS_THR * (single(time_since_trans_start_) / VT_PSHER_RMP_DT);
    | end
    | 
    | %% 如果提供了融合的airspeed,并通过了最小的转换时间,则将mc和fw控制融合在一起
    | % do blending of mc and fw controls if a blending airspeed has been provided and the minimum transition time has passed
    | % VT_ARSP_TRANS, 可以转换到固定翼模式时候的空速，默认10ms/s
    | % VT_ARSP_BLEND, 大于该值，可以融合fw controls和mc controls，默认8m/s
    | airspeed_trans_blend_margin = VT_ARSP_TRANS - VT_ARSP_BLEND;
    | 
    | if ((airspeed_trans_blend_margin > 0.0) && ...
    |         (isfinite(airspeed_validated.calibrated_airspeed_m_s)) && ...
    |         (airspeed_validated.calibrated_airspeed_m_s > 0.0) && ...
    |         (airspeed_validated.calibrated_airspeed_m_s >= VT_ARSP_BLEND) && ...
    |         (time_since_trans_start_ > VT_TRANS_MIN_TM))
    |     
    |     mc_weight_ = 1.0 - abs(airspeed_validated.calibrated_airspeed_m_s - VT_ARSP_BLEND) / airspeed_trans_blend_margin;
    |     
    | elseif (~isfinite(airspeed_validated.calibrated_airspeed_m_s))
    |     
    |     mc_weight_ = 1.0 - time_since_trans_start_ / VT_TRANS_MIN_TM;
    |     mc_weight_ = constrain(2.0 * mc_weight_, 0.0, 1.0);
    |     
    | end
    | 
    | % ramp up FW_PSP_OFF
    | vtol_att_sp.pitch_body = FW_PSP_OFF * (1.0 - mc_weight_);
    | vtol_att_sp.roll_body = fw_virtual_att_sp.roll_body;
    | 
    | % in stabilized, acro or manual mode, set the MC thrust to the throttle stick position (coming from the FW attitude setpoint)
    | % thrust_body: Normalized thrust command in body NED frame [-1,1];
    | if (~control_mode.flag_control_climb_rate_enabled)
    |     vtol_att_sp.thrust_body(3) = -fw_virtual_att_sp.thrust_body(1);
    | end
    | 
    | % 欧拉角到四元数
    | vtol_att_sp.q_d = euler2quat(vtol_att_sp.roll_body, vtol_att_sp.pitch_body, vtol_att_sp.yaw_body);
    | 
    | % check front transition timeout
    | % 检查前向转换是否超时
    | if ((VT_TRANS_TIMEOUT > eps) && (time_since_trans_start_ > VT_TRANS_TIMEOUT))
    |     % transition timeout occured, abort transition
    |     sprintf("Transition timeout")
    | end
    | 
    | end
  function transition_to_mc:
    | % Parameters
    | %% Delay in seconds before applying back transition throttle
    | % Set this to a value greater than 0 to give the motor time to spin down.
    | % unit s
    | % @min 0
    | % @max 10
    | % @increment 1
    | % @decimal 2
    | % @group VTOL Attitude Control
    | % PARAM_DEFINE_FLOAT(VT_B_REV_DEL, 0.0f);
    | 
    | %% Back transition MC motor ramp up time
    | % This sets the duration during which the MC motors ramp up to the commanded thrust during the back transition stage.
    | % @unit s
    | % @min 0.0
    | % @max 20.0
    | % @group VTOL Attitude Control
    | % PARAM_DEFINE_FLOAT(VT_B_TRANS_RAMP, 3.0f);
    | 
    | %% Approximate deceleration during back transition
    | % The approximate deceleration during a back transition in m/s/s
    | % Used to calculate back transition distance in mission mode. A lower value will make the VTOL transition further from the destination waypoint.
    | % For standard vtol and tiltrotors a controller is used to track this value during the transition.
    | % @unit m/s^2
    | % @min 0.5
    | % @max 10
    | % @increment 0.1
    | % @decimal 2
    | % @group VTOL Attitude Control
    | % PARAM_DEFINE_FLOAT(VT_B_DEC_MSS, 2.0f);
    | 
    | %% Backtransition deceleration setpoint to pitch feedforward gain.
    | % @unit rad s^2/m
    | % @min 0
    | % @max 0.2
    | % @decimal 1
    | % @increment 0.05
    | % @group VTOL Attitude Control
    | % PARAM_DEFINE_FLOAT(VT_B_DEC_FF, 0.12f);
    | 
    | %% 固定翼转多旋翼
    | function transition_to_mc
    | 
    | vtol_att_sp.roll_body = fw_virtual_att_sp.roll_body;
    | 
    | if (control_mode.flag_control_climb_rate_enabled)
    |     % control backtransition deceleration using pitch.
    |     vtol_att_sp.pitch_body = update_and_get_backtransition_pitch_sp();
    | end
    | 
    | % in stabilized, acro or manual mode, set the MC thrust to the throttle stick position (coming from the FW attitude setpoint)
    | if (~control_mode.flag_control_climb_rate_enabled)
    |     vtol_att_sp.thrust_body(3) = fw_virtual_att_sp.thrust_body(1);
    | end
    | 
    | % 四元数
    | vtol_att_sp.q_d = euler2quat(vtol_att_sp.roll_body, vtol_att_sp.pitch_body, vtol_att_sp.yaw_body);
    | 
    | pusher_throttle_ = single(0.0);
    | 
    | if (time_since_trans_start_ > VT_B_REV_DEL)
    |     % 减小油门用于刹车
    |     thrscale = (time_since_trans_start_ - VT_B_REV_DEL) / VT_PSHER_RMP_DT;
    |     thrscale = constrain(thrscale, 0.0, 1.0);
    |     pusher_throttle_ = thrscale * VT_B_TRANS_RAMP;
    | end
    | 
    | % continually increase mc attitude control as we transition back to mc mode
    | % 持续增加多旋翼控制的比例
    | if (VT_B_TRANS_RAMP > eps)
    |     mc_weight_ = time_since_trans_start_ / VT_B_TRANS_RAMP;
    | end
    | 
    | %% 设置电机状态
    | % set_all_motor_state(PX4_MOTOR_STATE.ENABLED, 0);
    | 
    | % set idle speed for MC actuators
    | % 保护
    | if(~flag_idle_mc_)
    | %    flag_idle_mc = set_idle_mc();
    | end
    | 
    | mc_weight_ = constrain(mc_weight_, 0.0, 1.0);
    | mc_roll_weight_ = mc_weight_;
    | mc_pitch_weight_ = mc_weight_;
    | mc_yaw_weight_ = mc_weight_;
    | mc_throttle_weight_ = mc_weight_;
    | 
    | end
    | 
    | %% 计算固定翼转旋翼，减速过渡期间的pitch_body
    | function pitch_body = update_and_get_backtransition_pitch_sp()
    | 
    | % 计算dt
    | persistent last_loop_ts;
    | if (isempty(last_loop_ts))
    |     last_loop_ts = single(0.0); % 单位：s
    | end
    | now = single(getSimulationTime);
    | transition_dt_ = (now - last_loop_ts); % 单位：s
    | last_loop_ts = now;
    | 
    | % maximum up or down pitch the controller is allowed to demand
    | pitch_lim = single(0.3);
    | euler = quat2eul(vehicle_att.q','ZYZ');
    | 
    | crack = atan2(local_pos.vy, local_pos.vx);
    | accel_body_forward = cos(crack) * local_pos.ax + sin(crack) * local_pos.ay;
    | 
    | % get accel error, positive means decelerating too slow, need to pitch up (must reverse dec_max, as it is a positive number)
    | accel_error_forward = VT_B_DEC_MSS + accel_body_forward;
    | 
    | pitch_sp_new = VT_B_DEC_FF * VT_B_DEC_MSS + accel_to_pitch_integ_;
    | 
    | integrator_input = VT_B_DEC_I * accel_error_forward;
    | 
    | % 防积分饱和
    | if ((pitch_sp_new >= pitch_lim && accel_error_forward > 0.0) || ...
    |         (pitch_sp_new <= -pitch_lim && accel_error_forward < 0.0))
    |     integrator_input = single(0.0);
    | end
    | 
    | accel_to_pitch_integ_ = accel_to_pitch_integ_ + integrator_input * transition_dt_;
    | 
    | pitch_body = constrain(pitch_sp_new, -pitch_lim, pitch_lim);
    | 
    | end
